simulink model "WindTurbineDrivelineWithVibrations"  (R2023a)
settings: Solver=ode23t  StartTime=0.0  StopTime=scenario.tEnd  MaxStep=2  RelTol=1e-3  AbsTol=1e-3
PreLoadFcn:
  | addpath('Libraries', 'Scripts_Data', 'Images');
model workspace: external: MATLAB File WindTurbineDrivelineWithVibrationsParameters.m (data not in the file)
undefined symbols (not defined in the file): Bampton, Craig, diff, fs, fsCB, m, N, rotor, scenario
libraries: fl_lib x33, nesl_utility x6, simulink x4, sdl_lib x3, slpidlib x1, nesl_utility_internal x1
(part 2 of 2)

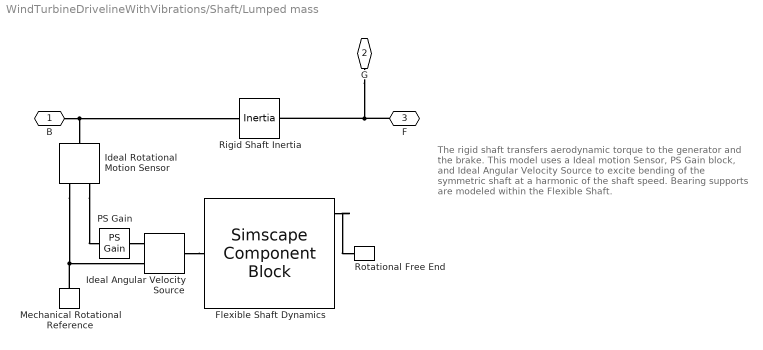
== system WindTurbineDrivelineWithVibrations/Shaft/Lumped mass ==
  note: The rigid shaft transfers aerodynamic torque to the generator and the brake.
      |
      | This model uses a Ideal motion Sensor, PS Gain block, and Ideal Angular Velocity Source to excite bending of the symmetric shaft at a harmonic of the shaft speed. Bearing supports are modeled within the Flexible Shaft.
  Flexible Shaft Dynamics : SimscapeComponentBlock  SourceFile=sdl.couplings.flexible_shaft  ComponentPath=sdl.couplings.flexible_shaft  ComponentVariants="[\"sdl.couplings.flexible_shaft\"]"  ComponentVariantNames="[\"flexible_shaft\"]"  ClassName=flexible_shaft  SchemaVersion=1  modelTorsion=true  modelTransverse=true  n_segments=1  parameterization=sdl.enum.shaftParameterization.MaterialPropertiesVaried  length=fs.length_shaft m  lengths=diff(fs.z_shaft) m  shaft_stiffness=2e5 N*m/rad  shaft_inertia=0.02 kg*m^2  shaft_stiffnesses=[400000, 200000, 100000] N*m/rad  shaft_inertias=[.025, .02, .015] kg*m^2  eiIN=5e5 Pa*m^4  rhoaIN=19 kg/m  eiINs=[600000, 500000, 400000] Pa*m^4  rhoaINs=[20, 19, 18] kg/m  density=fs.material_density kg/m^3  shear_modulus=fs.shear_modulus Pa  elastic_modulus=fs.elastic_modulus Pa  shaft_construction=sdl.enum.shaftConstruction.annular  diameter_outer=fs.diameters_outer(1) m  diameter_inner=fs.diameters_inner(1) m  diameter_outers=interp1(fs.z_TLU, fs.diameters_outer_TLU, fs.z_shaft(2:end)) m  diameter_inners=interp1(fs.z_TLU, fs.diameters_inner_TLU, fs.z_shaft(2:end)) m  damping_ratio=0.01  mu_visc_BF=[0, 0] N*m/(rad/s)  mu_visc=fs.mu_visc_tors N*m/(rad/s)  initial_deflection=0 rad  initial_velocity=0 rpm  num_supports=sdl.enum.num_supports.four  z_support=fs.z_support m  boundaryB1=sdl.enum.shaftSupport.bearingMatrix_speed  DrotB1_row=fs.bearing.d_rot N*m/(rad/s)  DtransB1_row=[20000, -44000, -44000, 350000] N/(m/s)  DtransB1_w_mat=fs.bearing.D N/(m/s)  KrotB1_row=fs.bearing.k_rot N*m/rad  KtransB1_row=[1000000, -200000, -300000, 5000000] N/m  KtransB1_w_mat=fs.bearing.K N/m  boundaryI1=sdl.enum.shaftSupport.bearingMatrix_speed  DrotI1_row=fs.bearing.d_rot N*m/(rad/s)  DtransI1_row=[20000, -44000, -44000, 350000] N/(m/s)  DtransI1_w_mat=fs.bearing.D N/(m/s)  KrotI1_row=fs.bearing.k_rot N*m/rad  KtransI1_row=[1000000, -200000, -300000, 5000000] N/m  KtransI1_w_mat=fs.bearing.K N/m  boundaryI2=sdl.enum.shaftSupport.bearingMatrix_speed  DrotI2_row=fs.bearing.d_rot N*m/(rad/s)  DtransI2_row=[20000, -44000, -44000, 350000] N/(m/s)  DtransI2_w_mat=fs.bearing.D N/(m/s)  KrotI2_row=fs.bearing.k_rot N*m/rad  KtransI2_row=[1000000, -200000, -300000, 5000000] N/m  KtransI2_w_mat=fs.bearing.K N/m  boundaryF1=sdl.enum.shaftSupport.bearingMatrix_speed  DrotF1_row=fs.bearing.d_rot N*m/(rad/s)  DtransF1_row=[20000, -44000, -44000, 350000] N/(m/s)  DtransF1_w_mat=fs.bearing.D N/(m/s)  KrotF1_row=fs.bearing.k_rot N*m/rad  KtransF1_row=[1000000, -200000, -300000, 5000000] N/m  KtransF1_w_mat=fs.bearing.K N/m  bearing_speed=fs.bearing_speed*fs.excitationPoles rpm  alpha=fs.a_damp 1/s  beta=fs.b_damp s  noDisk=sdl.enum.shaftDisks.disk  zDisk=fs.z_mass m  mDiskIN=fs.point_mass kg  IdDiskIN=fs.Id kg*m^2  IpDiskIN=fs.Ip./fs.excitationPoles kg*m^2  enable_static_unbalance=true  offsetMR=fs.excitationLoad./(fs.excitationPoles*fs.wNominal_forcing)^2 kg*m  offsetMR_initialAngleIN=0 rad  offsetMassLocation=fs.z_generator m  enable_external_force=false  externalForce=[1, 2] N  externalForceHarmonic=[.5, 2]  externalLoadAngle=[pi / 2, 3 * pi / 4] rad  zExternalLoad=[.25, .75] m  AnalysisMethod=sdl.enum.bendingAnalysisMethod.LumpedMass  ModeInputMethod=sdl.enum.modeInputMethod.SimscapeDetermined  numModesIn=fs.num_modes  mode_speed_dependency=sdl.enum.mode_speed_dependency.Dynamic  OmegaNom=fs.w_shaft_nominal rad/s  wMax=fs.wMax rad/s  dz=fs.dz m  userMode_w=[280, 644, 615, 1285] rad/s  userMode_w_mat=[257, 780, 580, 1560; 280, 644, 615, 1285; 294, 513, 636, 1020] rad/s  userMode_z=[0, .1, .2, .3, .4, .5, .6, .7, .8, .9, 1] m  userMode_shapeX=[.1648, .0086, -.2759, .0162; .1671, .0093, -.2231, .0133; .1691, .01, -.1689, .0102; .1707, .0105, -.1135, .007; .1717, .0108, -.057, .0035; .1721, .0109, 0, 0; .1717, .0108, .057, -.0035; .1707, .0105, .1135, -.007; .1691, .01, .1689, -.0102; .1671, .0093, .2231, -.0133; .1648, .0086, .2759, -.0162]  userMode_shapeX_mat=cat(3, [.1842, .0134, -.3072, .0272; .1863, .0152, -.2482, .0226; .1882, .0169, -.1878, .0176; .1897, .0182, -.1261, .0121; .1906, .019, -.0634, .0062; .191, .0193, 0, 0; .1906, .019, .0634, -.0062; .1897, .0182, .1261, -.0121; .1882, .0169, .1878, -.0176; .1863, .0152, .2482, -.0226; .1842, .0134, .3072, -.0272], [.1648, .0086, -.2759, .0162; .1671, .0093, -.2231, .0133; .1691, .01, -.1689, .0102; .1707, .0105, -.1135, .007; .1717, .0108, -.057, .0035; .1721, .0109, 0, 0; .1717, .0108, .057, -.0035; .1707, .0105, .1135, -.007; .1691, .01, .1689, -.0102; .1671, .0093, .2231, -.0133; .1648, .0086, .2759, -.0162], [.1291, .0046, -.2166, .0082; .131, .0048, -.1751, .0067; .1327, .005, -.1327, .0051; .1341, .0052, -.0891, .0035; .135, .0053, -.0448, .0017; .1353, .0053, 0, 0; .135, .0053, .0448, -.0017; .1341, .0052, .0891, -.0035; .1327, .005, .1327, -.0051; .131, .0048, .1751, -.0067; .1291, .0046, .2166, -.0082])  userMode_shapeY=[.1193, -.1784, -.1997, -.3348; .1209, -.1933, -.1615, -.2751; .1224, -.2068, -.1223, -.2119; .1235, -.2176, -.0821, -.1445; .1243, -.2245, -.0413, -.0734; .1246, -.2269, 0, 0; .1243, -.2245, .0413, .0734; .1235, -.2176, .0821, .1445; .1224, -.2068, .1223, .2119; .1209, -.1933, .1615, .2751; .1193, -.1784, .1997, .3348]  userMode_shapeY_mat=cat(3, [.0885, -.1625, -.1475, -.3301; .0895, -.1847, -.1192, -.2745; .0904, -.2048, -.0902, -.2141; .0911, -.2209, -.0606, -.1475; .0916, -.2313, -.0304, -.0754; .0917, -.2349, 0, 0; .0916, -.2313, .0304, .0754; .0911, -.2209, .0606, .1475; .0904, -.2048, .0902, .2141; .0895, -.1847, .1192, .2745; .0885, -.1625, .1475, .3301], [.1193, -.1784, -.1997, -.3348; .1209, -.1933, -.1615, -.2751; .1224, -.2068, -.1223, -.2119; .1235, -.2176, -.0821, -.1445; .1243, -.2245, -.0413, -.0734; .1246, -.2269, 0, 0; .1243, -.2245, .0413, .0734; .1235, -.2176, .0821, .1445; .1224, -.2068, .1223, .2119; .1209, -.1933, .1615, .2751; .1193, -.1784, .1997, .3348], [.1566, -.1901, -.2628, -.3377; .1589, -.1994, -.2125, -.2753; .161, -.2079, -.1609, -.2103; .1627, -.2146, -.1081, -.1424; .1638, -.219, -.0544, -.0719; .1642, -.2205, 0, 0; .1638, -.219, .0544, .0719; .1627, -.2146, .1081, .1424; .161, -.2079, .1609, .2103; .1589, -.1994, .2125, .2753; .1566, -.1901, .2628, .3377])  eta_lumped_nominal=1  etaDer_lumped_nominal=1  eta_modal_nominal=1  etaDer_modal_nominal=1
      settings: CopyFcn=simscape.engine.sli.internal.componentblockcallback(gcbh,'COPY')  PreCopyFcn=simscape.engine.sli.internal.componentblockcallback(gcbh,'PRECOPY')  PreDeleteFcn=simscape.engine.sli.internal.componentblockcallback(gcbh,'PREDELETE')  InternalSimscapePortConfiguration="{\"Bottom\":[{\"id\":\"Fsupports\",\"label\":\"Fr\",\"type\":\"output\"},{\"id\":\"Msupports\",\"label\":\"M\",\"type\":\"output\"},{\"id\":\"Vsupports\",\"label\":\"V\",\"type\":\"output\"},{\"id\":\"Wsupports\",\"label\":\"W\",\"type\":\"output\"}],\"Left\":[{\"id\":\"B\",\"label\":\"B\",\"type\":\"foundation.mechanical.rotational.rotational\"}],\"Right\":[{\"id\":\"F\",\"label\":\"F\",\"type\":\"foundation.mechanical.rotational.rotational\"}],\"Top\":[]}"
      mask Type: Flexible Shaft
  Ideal Angular Velocity Source : fl_lib/Mechanical/Mechanical Sources/Ideal Angular Velocity Source
  Ideal Rotational Motion Sensor : fl_lib/Mechanical/Mechanical Sensors/Ideal Rotational Motion Sensor  reference=foundation.enum.MeasurementReference.difference  acceleration_port=false  velocity_port=true  position_port=false  wrap_angle=false  offset=0 rad
      settings: InternalSimscapePortConfiguration="{\"Bottom\":[],\"Left\":[{\"id\":\"R\",\"label\":\"R\",\"type\":\"foundation.mechanical.rotational.rotational\"}],\"Right\":[{\"id\":\"C\",\"label\":\"C\",\"type\":\"foundation.mechanical.rotational.rotational\"},{\"id\":\"W\",\"label\":\"W\",\"type\":\"output\"}],\"Top\":[]}"
  Mechanical Rotational Reference : fl_lib/Mechanical/Rotational Elements/Mechanical Rotational Reference
  PS Gain : fl_lib/Physical Signals/Functions/PS Gain  gain=fs.excitationPoles
  Rigid Shaft Inertia : fl_lib/Mechanical/Rotational Elements/Inertia  inertia=fs.Ip_total kg*m^2  num_ports=foundation.enum.numPorts2.two  w_specify=off  w_priority=High  w=0 rad/s  w_nominal_specify=off  w_nominal_unit=rad/s  w_nominal_value=1  t_specify=off  t_priority=None  t=0 N*m  t_nominal_specify=off  t_nominal_unit=N*m  t_nominal_value=1
      settings: InternalSimscapePortConfiguration="{\"Bottom\":[],\"Left\":[{\"id\":\"I\",\"label\":\"\",\"type\":\"foundation.mechanical.rotational.rotational\"}],\"Right\":[{\"id\":\"J\",\"label\":\"\",\"type\":\"foundation.mechanical.rotational.rotational\"}],\"Top\":[]}"
  Rotational Free End : fl_lib/Mechanical/Rotational Elements/Rotational Free End  w_specify=off  w_priority=None  w=0 rad/s  w_nominal_specify=off  w_nominal_unit=rad/s  w_nominal_value=1
  B : PMIOPort  Side=Left
  G : PMIOPort  Port=2  Side=Left
  F : PMIOPort  Port=3  Side=Right
  connections:
  F/RConn1 -- Rigid Shaft Inertia/LConn1 -- G/RConn1
  B/RConn1 -- Rigid Shaft Inertia/RConn1 -- Ideal Rotational Motion Sensor/LConn1
  Mechanical Rotational Reference/LConn1 -- Ideal Angular Velocity Source/RConn2 -- Ideal Rotational Motion Sensor/RConn1
  Ideal Angular Velocity Source/LConn1 -- Flexible Shaft Dynamics/LConn1
  PS Gain/RConn1 -- Ideal Angular Velocity Source/RConn1
  Ideal Rotational Motion Sensor/RConn2 -- PS Gain/LConn1
  Flexible Shaft Dynamics/RConn1 -- Rotational Free End/LConn1

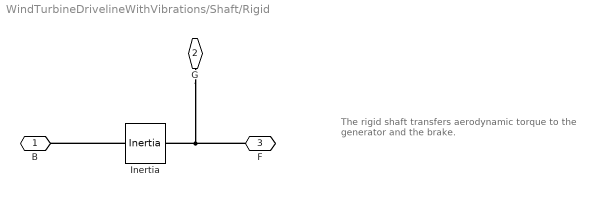
== system WindTurbineDrivelineWithVibrations/Shaft/Rigid ==
  note: The rigid shaft transfers aerodynamic torque to the generator and the brake.
  Inertia : fl_lib/Mechanical/Rotational Elements/Inertia  inertia=fs.Ip_total kg*m^2  num_ports=foundation.enum.numPorts2.two  w_specify=off  w_priority=High  w=0 rad/s  w_nominal_specify=off  w_nominal_unit=rad/s  w_nominal_value=1  t_specify=off  t_priority=None  t=0 N*m  t_nominal_specify=off  t_nominal_unit=N*m  t_nominal_value=1
      settings: InternalSimscapePortConfiguration="{\"Bottom\":[],\"Left\":[{\"id\":\"I\",\"label\":\"\",\"type\":\"foundation.mechanical.rotational.rotational\"}],\"Right\":[{\"id\":\"J\",\"label\":\"\",\"type\":\"foundation.mechanical.rotational.rotational\"}],\"Top\":[]}"
  B : PMIOPort  Side=Left
  G : PMIOPort  Port=2  Side=Left
  F : PMIOPort  Port=3  Side=Right
  connections:
  Inertia/RConn1 -- B/RConn1
  F/RConn1 -- G/RConn1 -- Inertia/LConn1

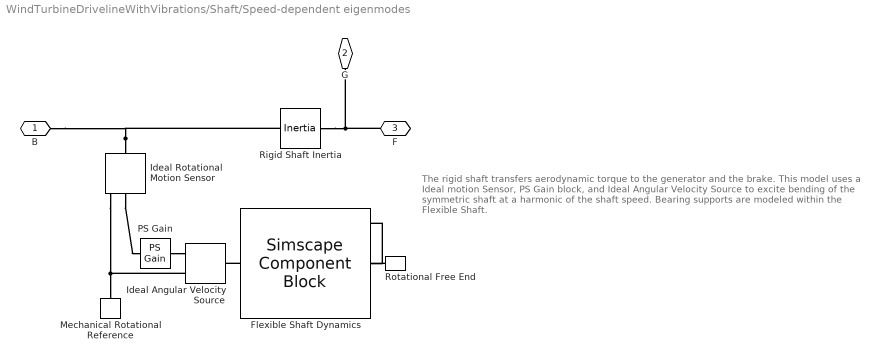
== system WindTurbineDrivelineWithVibrations/Shaft/Speed-dependent eigenmodes ==
  note: The rigid shaft transfers aerodynamic torque to the generator and the brake.
      |
      | This model uses a Ideal motion Sensor, PS Gain block, and Ideal Angular Velocity Source to excite bending of the symmetric shaft at a harmonic of the shaft speed. Bearing supports are modeled within the Flexible Shaft.
  Flexible Shaft Dynamics : SimscapeComponentBlock  SourceFile=sdl.couplings.flexible_shaft  ComponentPath=sdl.couplings.flexible_shaft  ComponentVariants="[\"sdl.couplings.flexible_shaft\"]"  ComponentVariantNames="[\"flexible_shaft\"]"  ClassName=flexible_shaft  SchemaVersion=1  modelTorsion=true  modelTransverse=true  n_segments=1  parameterization=sdl.enum.shaftParameterization.MaterialPropertiesVaried  length=fs.length_shaft m  lengths=diff(fs.z_shaft) m  shaft_stiffness=2e5 N*m/rad  shaft_inertia=0.02 kg*m^2  shaft_stiffnesses=[400000, 200000, 100000] N*m/rad  shaft_inertias=[.025, .02, .015] kg*m^2  eiIN=5e5 Pa*m^4  rhoaIN=19 kg/m  eiINs=[600000, 500000, 400000] Pa*m^4  rhoaINs=[20, 19, 18] kg/m  density=fs.material_density kg/m^3  shear_modulus=fs.shear_modulus Pa  elastic_modulus=fs.elastic_modulus Pa  shaft_construction=sdl.enum.shaftConstruction.annular  diameter_outer=fs.diameters_outer(1) m  diameter_inner=fs.diameters_inner(1) m  diameter_outers=interp1(fs.z_TLU, fs.diameters_outer_TLU, fs.z_shaft(2:end)) m  diameter_inners=interp1(fs.z_TLU, fs.diameters_inner_TLU, fs.z_shaft(2:end)) m  damping_ratio=0.01  mu_visc_BF=[0, 0] N*m/(rad/s)  mu_visc=fs.mu_visc_tors N*m/(rad/s)  initial_deflection=0 rad  initial_velocity=0 rpm  num_supports=sdl.enum.num_supports.four  z_support=fs.z_support m  boundaryB1=sdl.enum.shaftSupport.bearingMatrix_speed  DrotB1_row=fs.bearing.d_rot N*m/(rad/s)  DtransB1_row=[20000, -44000, -44000, 350000] N/(m/s)  DtransB1_w_mat=fs.bearing.D N/(m/s)  KrotB1_row=fs.bearing.k_rot N*m/rad  KtransB1_row=[1000000, -200000, -300000, 5000000] N/m  KtransB1_w_mat=fs.bearing.K N/m  boundaryI1=sdl.enum.shaftSupport.bearingMatrix_speed  DrotI1_row=fs.bearing.d_rot N*m/(rad/s)  DtransI1_row=[20000, -44000, -44000, 350000] N/(m/s)  DtransI1_w_mat=fs.bearing.D N/(m/s)  KrotI1_row=fs.bearing.k_rot N*m/rad  KtransI1_row=[1000000, -200000, -300000, 5000000] N/m  KtransI1_w_mat=fs.bearing.K N/m  boundaryI2=sdl.enum.shaftSupport.bearingMatrix_speed  DrotI2_row=fs.bearing.d_rot N*m/(rad/s)  DtransI2_row=[20000, -44000, -44000, 350000] N/(m/s)  DtransI2_w_mat=fs.bearing.D N/(m/s)  KrotI2_row=fs.bearing.k_rot N*m/rad  KtransI2_row=[1000000, -200000, -300000, 5000000] N/m  KtransI2_w_mat=fs.bearing.K N/m  boundaryF1=sdl.enum.shaftSupport.bearingMatrix_speed  DrotF1_row=fs.bearing.d_rot N*m/(rad/s)  DtransF1_row=[20000, -44000, -44000, 350000] N/(m/s)  DtransF1_w_mat=fs.bearing.D N/(m/s)  KrotF1_row=fs.bearing.k_rot N*m/rad  KtransF1_row=[1000000, -200000, -300000, 5000000] N/m  KtransF1_w_mat=fs.bearing.K N/m  bearing_speed=fs.bearing_speed*fs.excitationPoles rpm  alpha=fs.a_damp 1/s  beta=fs.b_damp s  noDisk=sdl.enum.shaftDisks.disk  zDisk=fs.z_mass m  mDiskIN=fs.point_mass kg  IdDiskIN=fs.Id kg*m^2  IpDiskIN=fs.Ip./fs.excitationPoles kg*m^2  enable_static_unbalance=true  offsetMR=fs.excitationLoad./(fs.excitationPoles*fs.wNominal_forcing)^2 kg*m  offsetMR_initialAngleIN=0 rad  offsetMassLocation=fs.z_generator m  enable_external_force=false  externalForce=[1, 2] N  externalForceHarmonic=[.5, 2]  externalLoadAngle=[pi / 2, 3 * pi / 4] rad  zExternalLoad=[.25, .75] m  AnalysisMethod=sdl.enum.bendingAnalysisMethod.Eigenmodes  ModeInputMethod=sdl.enum.modeInputMethod.SimscapeDetermined  numModesIn=fs.num_modes  mode_speed_dependency=sdl.enum.mode_speed_dependency.Dynamic  OmegaNom=fs.w_shaft_nominal_static_eig rad/s  wMax=fs.wMax rad/s  dz=fs.dz m  userMode_w=[280, 644, 615, 1285] rad/s  userMode_w_mat=[257, 780, 580, 1560; 280, 644, 615, 1285; 294, 513, 636, 1020] rad/s  userMode_z=[0, .1, .2, .3, .4, .5, .6, .7, .8, .9, 1] m  userMode_shapeX=[.1648, .0086, -.2759, .0162; .1671, .0093, -.2231, .0133; .1691, .01, -.1689, .0102; .1707, .0105, -.1135, .007; .1717, .0108, -.057, .0035; .1721, .0109, 0, 0; .1717, .0108, .057, -.0035; .1707, .0105, .1135, -.007; .1691, .01, .1689, -.0102; .1671, .0093, .2231, -.0133; .1648, .0086, .2759, -.0162]  userMode_shapeX_mat=cat(3, [.1842, .0134, -.3072, .0272; .1863, .0152, -.2482, .0226; .1882, .0169, -.1878, .0176; .1897, .0182, -.1261, .0121; .1906, .019, -.0634, .0062; .191, .0193, 0, 0; .1906, .019, .0634, -.0062; .1897, .0182, .1261, -.0121; .1882, .0169, .1878, -.0176; .1863, .0152, .2482, -.0226; .1842, .0134, .3072, -.0272], [.1648, .0086, -.2759, .0162; .1671, .0093, -.2231, .0133; .1691, .01, -.1689, .0102; .1707, .0105, -.1135, .007; .1717, .0108, -.057, .0035; .1721, .0109, 0, 0; .1717, .0108, .057, -.0035; .1707, .0105, .1135, -.007; .1691, .01, .1689, -.0102; .1671, .0093, .2231, -.0133; .1648, .0086, .2759, -.0162], [.1291, .0046, -.2166, .0082; .131, .0048, -.1751, .0067; .1327, .005, -.1327, .0051; .1341, .0052, -.0891, .0035; .135, .0053, -.0448, .0017; .1353, .0053, 0, 0; .135, .0053, .0448, -.0017; .1341, .0052, .0891, -.0035; .1327, .005, .1327, -.0051; .131, .0048, .1751, -.0067; .1291, .0046, .2166, -.0082])  userMode_shapeY=[.1193, -.1784, -.1997, -.3348; .1209, -.1933, -.1615, -.2751; .1224, -.2068, -.1223, -.2119; .1235, -.2176, -.0821, -.1445; .1243, -.2245, -.0413, -.0734; .1246, -.2269, 0, 0; .1243, -.2245, .0413, .0734; .1235, -.2176, .0821, .1445; .1224, -.2068, .1223, .2119; .1209, -.1933, .1615, .2751; .1193, -.1784, .1997, .3348]  userMode_shapeY_mat=cat(3, [.0885, -.1625, -.1475, -.3301; .0895, -.1847, -.1192, -.2745; .0904, -.2048, -.0902, -.2141; .0911, -.2209, -.0606, -.1475; .0916, -.2313, -.0304, -.0754; .0917, -.2349, 0, 0; .0916, -.2313, .0304, .0754; .0911, -.2209, .0606, .1475; .0904, -.2048, .0902, .2141; .0895, -.1847, .1192, .2745; .0885, -.1625, .1475, .3301], [.1193, -.1784, -.1997, -.3348; .1209, -.1933, -.1615, -.2751; .1224, -.2068, -.1223, -.2119; .1235, -.2176, -.0821, -.1445; .1243, -.2245, -.0413, -.0734; .1246, -.2269, 0, 0; .1243, -.2245, .0413, .0734; .1235, -.2176, .0821, .1445; .1224, -.2068, .1223, .2119; .1209, -.1933, .1615, .2751; .1193, -.1784, .1997, .3348], [.1566, -.1901, -.2628, -.3377; .1589, -.1994, -.2125, -.2753; .161, -.2079, -.1609, -.2103; .1627, -.2146, -.1081, -.1424; .1638, -.219, -.0544, -.0719; .1642, -.2205, 0, 0; .1638, -.219, .0544, .0719; .1627, -.2146, .1081, .1424; .161, -.2079, .1609, .2103; .1589, -.1994, .2125, .2753; .1566, -.1901, .2628, .3377])  eta_lumped_nominal=1  etaDer_lumped_nominal=1  eta_modal_nominal=1  etaDer_modal_nominal=1
      settings: CopyFcn=simscape.engine.sli.internal.componentblockcallback(gcbh,'COPY')  PreCopyFcn=simscape.engine.sli.internal.componentblockcallback(gcbh,'PRECOPY')  PreDeleteFcn=simscape.engine.sli.internal.componentblockcallback(gcbh,'PREDELETE')  InternalSimscapePortConfiguration="{\"Bottom\":[{\"id\":\"Fsupports\",\"label\":\"Fr\",\"type\":\"output\"},{\"id\":\"Msupports\",\"label\":\"M\",\"type\":\"output\"},{\"id\":\"Vsupports\",\"label\":\"V\",\"type\":\"output\"},{\"id\":\"Wsupports\",\"label\":\"W\",\"type\":\"output\"}],\"Left\":[{\"id\":\"B\",\"label\":\"B\",\"type\":\"foundation.mechanical.rotational.rotational\"}],\"Right\":[{\"id\":\"F\",\"label\":\"F\",\"type\":\"foundation.mechanical.rotational.rotational\"}],\"Top\":[]}"
      mask Type: Flexible Shaft
  Ideal Angular Velocity Source : fl_lib/Mechanical/Mechanical Sources/Ideal Angular Velocity Source
  Ideal Rotational Motion Sensor : fl_lib/Mechanical/Mechanical Sensors/Ideal Rotational Motion Sensor  reference=foundation.enum.MeasurementReference.difference  acceleration_port=false  velocity_port=true  position_port=true  wrap_angle=false  offset=0 rad
  Mechanical Rotational Reference : fl_lib/Mechanical/Rotational Elements/Mechanical Rotational Reference
  PS Gain : fl_lib/Physical Signals/Functions/PS Gain  gain=fs.excitationPoles
  Rigid Shaft Inertia : fl_lib/Mechanical/Rotational Elements/Inertia  inertia=fs.Ip_total kg*m^2  num_ports=foundation.enum.numPorts2.two  w_specify=off  w_priority=High  w=0 rad/s  w_nominal_specify=off  w_nominal_unit=rad/s  w_nominal_value=1  t_specify=off  t_priority=None  t=0 N*m  t_nominal_specify=off  t_nominal_unit=N*m  t_nominal_value=1
      settings: InternalSimscapePortConfiguration="{\"Bottom\":[],\"Left\":[{\"id\":\"I\",\"label\":\"\",\"type\":\"foundation.mechanical.rotational.rotational\"}],\"Right\":[{\"id\":\"J\",\"label\":\"\",\"type\":\"foundation.mechanical.rotational.rotational\"}],\"Top\":[]}"
  Rotational Free End : fl_lib/Mechanical/Rotational Elements/Rotational Free End  w_specify=off  w_priority=None  w=0 rad/s  w_nominal_specify=off  w_nominal_unit=rad/s  w_nominal_value=1
  B : PMIOPort  Side=Left
  G : PMIOPort  Port=2  Side=Left
  F : PMIOPort  Port=3  Side=Right
  connections:
  Ideal Rotational Motion Sensor/LConn1 -- Rigid Shaft Inertia/RConn1 -- B/RConn1
  Ideal Rotational Motion Sensor/RConn2 -- PS Gain/LConn1
  Flexible Shaft Dynamics/LConn1 -- Ideal Angular Velocity Source/LConn1
  PS Gain/RConn1 -- Ideal Angular Velocity Source/RConn1
  Rotational Free End/LConn1 -- Flexible Shaft Dynamics/RConn1
  Rigid Shaft Inertia/LConn1 -- G/RConn1 -- F/RConn1
  Ideal Rotational Motion Sensor/RConn1 -- Ideal Angular Velocity Source/RConn2 -- Mechanical Rotational Reference/LConn1

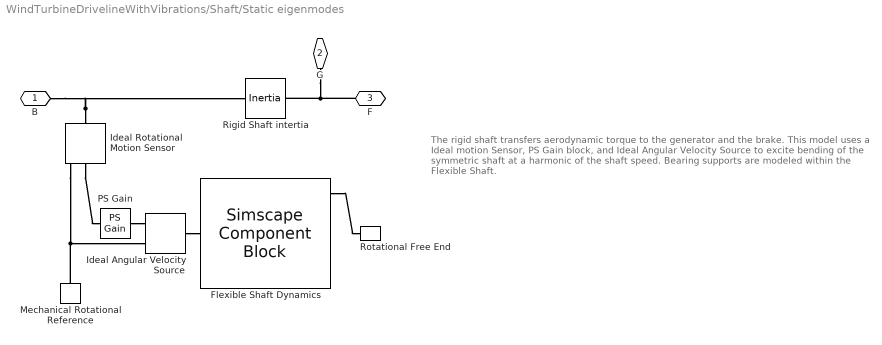
== system WindTurbineDrivelineWithVibrations/Shaft/Static eigenmodes ==
  note: The rigid shaft transfers aerodynamic torque to the generator and the brake.
      |
      | This model uses a Ideal motion Sensor, PS Gain block, and Ideal Angular Velocity Source to excite bending of the symmetric shaft at a harmonic of the shaft speed. Bearing supports are modeled within the Flexible Shaft.
  Flexible Shaft Dynamics : SimscapeComponentBlock  SourceFile=sdl.couplings.flexible_shaft  ComponentPath=sdl.couplings.flexible_shaft  ComponentVariants="[\"sdl.couplings.flexible_shaft\"]"  ComponentVariantNames="[\"flexible_shaft\"]"  ClassName=flexible_shaft  SchemaVersion=1  modelTorsion=true  modelTransverse=true  n_segments=1  parameterization=sdl.enum.shaftParameterization.MaterialPropertiesVaried  length=fs.length_shaft m  lengths=diff(fs.z_shaft) m  shaft_stiffness=2e5 N*m/rad  shaft_inertia=0.02 kg*m^2  shaft_stiffnesses=[400000, 200000, 100000] N*m/rad  shaft_inertias=[.025, .02, .015] kg*m^2  eiIN=5e5 Pa*m^4  rhoaIN=19 kg/m  eiINs=[600000, 500000, 400000] Pa*m^4  rhoaINs=[20, 19, 18] kg/m  density=fs.material_density kg/m^3  shear_modulus=fs.shear_modulus Pa  elastic_modulus=fs.elastic_modulus Pa  shaft_construction=sdl.enum.shaftConstruction.annular  diameter_outer=fs.diameters_outer(1) m  diameter_inner=fs.diameters_inner(1) m  diameter_outers=interp1(fs.z_TLU, fs.diameters_outer_TLU, fs.z_shaft(2:end)) m  diameter_inners=interp1(fs.z_TLU, fs.diameters_inner_TLU, fs.z_shaft(2:end)) m  damping_ratio=0.01  mu_visc_BF=[0, 0] N*m/(rad/s)  mu_visc=fs.mu_visc_tors N*m/(rad/s)  initial_deflection=0 rad  initial_velocity=0 rpm  num_supports=sdl.enum.num_supports.four  z_support=fs.z_support m  boundaryB1=sdl.enum.shaftSupport.bearingMatrix_speed  DrotB1_row=fs.bearing.d_rot N*m/(rad/s)  DtransB1_row=[20000, -44000, -44000, 350000] N/(m/s)  DtransB1_w_mat=fs.bearing.D N/(m/s)  KrotB1_row=fs.bearing.k_rot N*m/rad  KtransB1_row=[1000000, -200000, -300000, 5000000] N/m  KtransB1_w_mat=fs.bearing.K N/m  boundaryI1=sdl.enum.shaftSupport.bearingMatrix_speed  DrotI1_row=fs.bearing.d_rot N*m/(rad/s)  DtransI1_row=[20000, -44000, -44000, 350000] N/(m/s)  DtransI1_w_mat=fs.bearing.D N/(m/s)  KrotI1_row=fs.bearing.k_rot N*m/rad  KtransI1_row=[1000000, -200000, -300000, 5000000] N/m  KtransI1_w_mat=fs.bearing.K N/m  boundaryI2=sdl.enum.shaftSupport.bearingMatrix_speed  DrotI2_row=fs.bearing.d_rot N*m/(rad/s)  DtransI2_row=[20000, -44000, -44000, 350000] N/(m/s)  DtransI2_w_mat=fs.bearing.D N/(m/s)  KrotI2_row=fs.bearing.k_rot N*m/rad  KtransI2_row=[1000000, -200000, -300000, 5000000] N/m  KtransI2_w_mat=fs.bearing.K N/m  boundaryF1=sdl.enum.shaftSupport.bearingMatrix_speed  DrotF1_row=fs.bearing.d_rot N*m/(rad/s)  DtransF1_row=[20000, -44000, -44000, 350000] N/(m/s)  DtransF1_w_mat=fs.bearing.D N/(m/s)  KrotF1_row=fs.bearing.k_rot N*m/rad  KtransF1_row=[1000000, -200000, -300000, 5000000] N/m  KtransF1_w_mat=fs.bearing.K N/m  bearing_speed=fs.bearing_speed*fs.excitationPoles rpm  alpha=fs.a_damp 1/s  beta=fs.b_damp s  noDisk=sdl.enum.shaftDisks.disk  zDisk=fs.z_mass m  mDiskIN=fs.point_mass kg  IdDiskIN=fs.Id kg*m^2  IpDiskIN=fs.Ip./fs.excitationPoles kg*m^2  enable_static_unbalance=true  offsetMR=fs.excitationLoad./(fs.excitationPoles*fs.wNominal_forcing)^2 kg*m  offsetMR_initialAngleIN=0 rad  offsetMassLocation=fs.z_generator m  enable_external_force=false  externalForce=[1, 2] N  externalForceHarmonic=[.5, 2]  externalLoadAngle=[pi / 2, 3 * pi / 4] rad  zExternalLoad=[.25, .75] m  AnalysisMethod=sdl.enum.bendingAnalysisMethod.Eigenmodes  ModeInputMethod=sdl.enum.modeInputMethod.SimscapeDetermined  numModesIn=fs.num_modes  mode_speed_dependency=sdl.enum.mode_speed_dependency.Static  OmegaNom=fs.w_shaft_nominal_static_eig rad/s  wMax=fs.wMax rad/s  dz=fs.dz m  userMode_w=[280, 644, 615, 1285] rad/s  userMode_w_mat=[257, 780, 580, 1560; 280, 644, 615, 1285; 294, 513, 636, 1020] rad/s  userMode_z=[0, .1, .2, .3, .4, .5, .6, .7, .8, .9, 1] m  userMode_shapeX=[.1648, .0086, -.2759, .0162; .1671, .0093, -.2231, .0133; .1691, .01, -.1689, .0102; .1707, .0105, -.1135, .007; .1717, .0108, -.057, .0035; .1721, .0109, 0, 0; .1717, .0108, .057, -.0035; .1707, .0105, .1135, -.007; .1691, .01, .1689, -.0102; .1671, .0093, .2231, -.0133; .1648, .0086, .2759, -.0162]  userMode_shapeX_mat=cat(3, [.1842, .0134, -.3072, .0272; .1863, .0152, -.2482, .0226; .1882, .0169, -.1878, .0176; .1897, .0182, -.1261, .0121; .1906, .019, -.0634, .0062; .191, .0193, 0, 0; .1906, .019, .0634, -.0062; .1897, .0182, .1261, -.0121; .1882, .0169, .1878, -.0176; .1863, .0152, .2482, -.0226; .1842, .0134, .3072, -.0272], [.1648, .0086, -.2759, .0162; .1671, .0093, -.2231, .0133; .1691, .01, -.1689, .0102; .1707, .0105, -.1135, .007; .1717, .0108, -.057, .0035; .1721, .0109, 0, 0; .1717, .0108, .057, -.0035; .1707, .0105, .1135, -.007; .1691, .01, .1689, -.0102; .1671, .0093, .2231, -.0133; .1648, .0086, .2759, -.0162], [.1291, .0046, -.2166, .0082; .131, .0048, -.1751, .0067; .1327, .005, -.1327, .0051; .1341, .0052, -.0891, .0035; .135, .0053, -.0448, .0017; .1353, .0053, 0, 0; .135, .0053, .0448, -.0017; .1341, .0052, .0891, -.0035; .1327, .005, .1327, -.0051; .131, .0048, .1751, -.0067; .1291, .0046, .2166, -.0082])  userMode_shapeY=[.1193, -.1784, -.1997, -.3348; .1209, -.1933, -.1615, -.2751; .1224, -.2068, -.1223, -.2119; .1235, -.2176, -.0821, -.1445; .1243, -.2245, -.0413, -.0734; .1246, -.2269, 0, 0; .1243, -.2245, .0413, .0734; .1235, -.2176, .0821, .1445; .1224, -.2068, .1223, .2119; .1209, -.1933, .1615, .2751; .1193, -.1784, .1997, .3348]  userMode_shapeY_mat=cat(3, [.0885, -.1625, -.1475, -.3301; .0895, -.1847, -.1192, -.2745; .0904, -.2048, -.0902, -.2141; .0911, -.2209, -.0606, -.1475; .0916, -.2313, -.0304, -.0754; .0917, -.2349, 0, 0; .0916, -.2313, .0304, .0754; .0911, -.2209, .0606, .1475; .0904, -.2048, .0902, .2141; .0895, -.1847, .1192, .2745; .0885, -.1625, .1475, .3301], [.1193, -.1784, -.1997, -.3348; .1209, -.1933, -.1615, -.2751; .1224, -.2068, -.1223, -.2119; .1235, -.2176, -.0821, -.1445; .1243, -.2245, -.0413, -.0734; .1246, -.2269, 0, 0; .1243, -.2245, .0413, .0734; .1235, -.2176, .0821, .1445; .1224, -.2068, .1223, .2119; .1209, -.1933, .1615, .2751; .1193, -.1784, .1997, .3348], [.1566, -.1901, -.2628, -.3377; .1589, -.1994, -.2125, -.2753; .161, -.2079, -.1609, -.2103; .1627, -.2146, -.1081, -.1424; .1638, -.219, -.0544, -.0719; .1642, -.2205, 0, 0; .1638, -.219, .0544, .0719; .1627, -.2146, .1081, .1424; .161, -.2079, .1609, .2103; .1589, -.1994, .2125, .2753; .1566, -.1901, .2628, .3377])  eta_lumped_nominal=1  etaDer_lumped_nominal=1  eta_modal_nominal=1  etaDer_modal_nominal=1
      settings: CopyFcn=simscape.engine.sli.internal.componentblockcallback(gcbh,'COPY')  PreCopyFcn=simscape.engine.sli.internal.componentblockcallback(gcbh,'PRECOPY')  PreDeleteFcn=simscape.engine.sli.internal.componentblockcallback(gcbh,'PREDELETE')  InternalSimscapePortConfiguration="{\"Bottom\":[{\"id\":\"Fsupports\",\"label\":\"Fr\",\"type\":\"output\"},{\"id\":\"Msupports\",\"label\":\"M\",\"type\":\"output\"},{\"id\":\"Vsupports\",\"label\":\"V\",\"type\":\"output\"},{\"id\":\"Wsupports\",\"label\":\"W\",\"type\":\"output\"}],\"Left\":[{\"id\":\"B\",\"label\":\"B\",\"type\":\"foundation.mechanical.rotational.rotational\"}],\"Right\":[{\"id\":\"F\",\"label\":\"F\",\"type\":\"foundation.mechanical.rotational.rotational\"}],\"Top\":[]}"
      mask Type: Flexible Shaft
  Ideal Angular Velocity Source : fl_lib/Mechanical/Mechanical Sources/Ideal Angular Velocity Source
  Ideal Rotational Motion Sensor : fl_lib/Mechanical/Mechanical Sensors/Ideal Rotational Motion Sensor  reference=foundation.enum.MeasurementReference.difference  acceleration_port=false  velocity_port=true  position_port=true  wrap_angle=false  offset=0 rad
  Mechanical Rotational Reference : fl_lib/Mechanical/Rotational Elements/Mechanical Rotational Reference
  PS Gain : fl_lib/Physical Signals/Functions/PS Gain  gain=fs.excitationPoles
  Rigid Shaft intertia : fl_lib/Mechanical/Rotational Elements/Inertia  inertia=fs.Ip_total kg*m^2  num_ports=foundation.enum.numPorts2.two  w_specify=off  w_priority=High  w=0 rad/s  w_nominal_specify=off  w_nominal_unit=rad/s  w_nominal_value=1  t_specify=off  t_priority=None  t=0 N*m  t_nominal_specify=off  t_nominal_unit=N*m  t_nominal_value=1
      settings: InternalSimscapePortConfiguration="{\"Bottom\":[],\"Left\":[{\"id\":\"I\",\"label\":\"\",\"type\":\"foundation.mechanical.rotational.rotational\"}],\"Right\":[{\"id\":\"J\",\"label\":\"\",\"type\":\"foundation.mechanical.rotational.rotational\"}],\"Top\":[]}"
  Rotational Free End : fl_lib/Mechanical/Rotational Elements/Rotational Free End  w_specify=off  w_priority=None  w=0 rad/s  w_nominal_specify=off  w_nominal_unit=rad/s  w_nominal_value=1
  B : PMIOPort  Side=Left
  G : PMIOPort  Port=2  Side=Left
  F : PMIOPort  Port=3  Side=Right
  connections:
  Ideal Angular Velocity Source/LConn1 -- Flexible Shaft Dynamics/LConn1
  F/RConn1 -- G/RConn1 -- Rigid Shaft intertia/LConn1
  Ideal Rotational Motion Sensor/LConn1 -- B/RConn1 -- Rigid Shaft intertia/RConn1
  Ideal Rotational Motion Sensor/RConn2 -- PS Gain/LConn1
  PS Gain/RConn1 -- Ideal Angular Velocity Source/RConn1
  Flexible Shaft Dynamics/RConn1 -- Rotational Free End/LConn1
  Mechanical Rotational Reference/LConn1 -- Ideal Rotational Motion Sensor/RConn1 -- Ideal Angular Velocity Source/RConn2
